simulink model "TodoModelo"  (R2020b)
settings: Solver=VariableStepAuto  StartTime=0.0  StopTime=10.0  RelTol=1e-3
values from neighbouring files (symbols this model uses):
  delay = exp(-ts*s/2)    [ControlP.m]
  Fa = tf(1,1)    [ControlP.m]
  K = mu*Kp    [ControlP.m]    (also in ControlPID_RF.m)
  P = Km/(Tm*s+1)/(Tf*s+1)    [ControlP.m]    (also in ControlPID_RF.m)
  Pd = c2d(P,ts)    [ControlP.m]    (also in ControlPID_RF.m = -P)
  ts = 0.005    [ControlP.m]    (also in ControlPID_RF.m; DatosIdentVel_rampa.mat)
  Ts = ts    (= 0.005)    [ControlP.m]
settings Model: Creator=Fran  LastModifiedBy=Fran

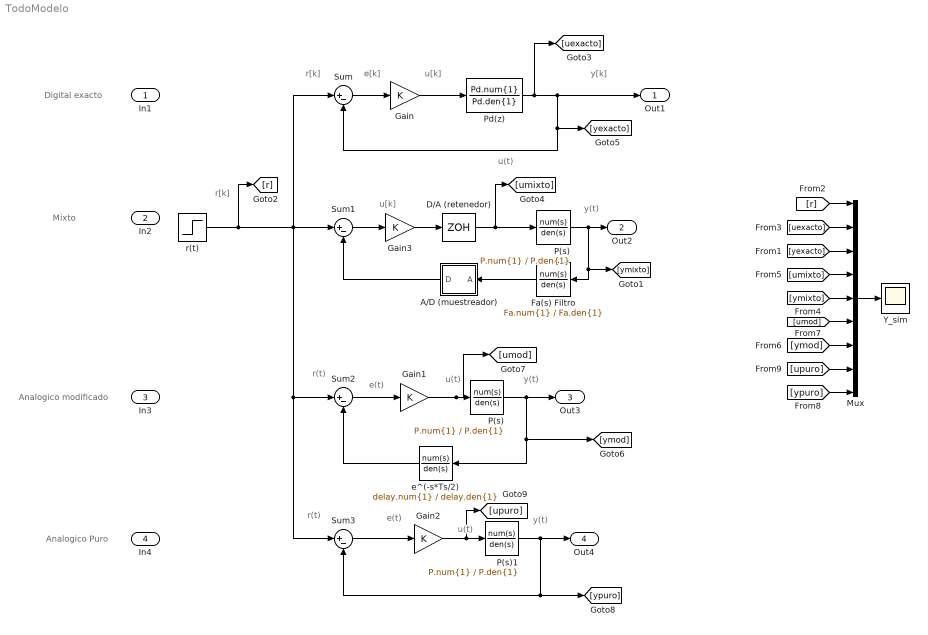
== system TodoModelo ==
  note: Analogico Puro
  note: Analogico modificado
  note: Mixto
  note: Digital exacto
  note: e[k]
  note: r[k]
  note: y[k]
  note: u[k]
  note: y(t)
  note: u[k]
  note: r[k]
  note: u(t)
  note: u(t)
  note: r(t)
  note: y(t)
  note: e(t)
  note: y(t)
  note: r(t)
  note: u(t)
  note: e(t)
  In1 : Inport
  In2 : Inport  Port=2
  In3 : Inport  Port=3
  In4 : Inport  Port=4
  A/D (muestreador) : Subsystem
  D/A (retenedor) : ZeroOrderHold  SampleTime=ts
  Fa(s) Filtro : TransferFcn  Numerator=Fa.num{1}  Denominator=Fa.den{1}
  Gain{,1..3} (4 alike) : Gain  Gain=K
  Mux : Mux  Inputs=9
  P(s) : TransferFcn  Numerator=P.num{1}  Denominator=P.den{1}
  "P(s) " : TransferFcn  Numerator=P.num{1}  Denominator=P.den{1}
  P(s)1 : TransferFcn  Numerator=P.num{1}  Denominator=P.den{1}
  Pd(z) : DiscreteTransferFcn  Numerator=Pd.num{1}  Denominator=Pd.den{1}  SampleTime=Ts
  Sum{,1..3} (4 alike) : Sum  Inputs=|+-
  Y_sim : Scope
  e^(-s*Ts/2) : TransferFcn  Numerator=delay.num{1}  Denominator=delay.den{1}
  r(t) : Step  SampleTime=ts
  Out1 : Outport
  Out2 : Outport  Port=2
  Out3 : Outport  Port=3
  Out4 : Outport  Port=4
  wires:
  Sum/1 -> Gain/1
  Gain/1 -> Pd(z)/1
  Mux/1 -> Y_sim/1
  Fa(s) Filtro/1 -> A/D (muestreador)/1(A)
  D/A (retenedor)/1 -> [umixto], "P(s) "/1
  [r] -> Mux/1
  "P(s) "/1 -> Fa(s) Filtro/1, [ymixto], Out2/1
  r(t)/1 -> Sum1/1, Sum/1, Sum3/1, Sum2/1, [r]
  [yexacto] -> Mux/3
  [uexacto] -> Mux/2
  Sum2/1 -> Gain1/1
  e^(-s*Ts/2)/1 -> Sum2/2
  P(s)/1 -> [ymod], e^(-s*Ts/2)/1, Out3/1
  Gain1/1 -> [umod], P(s)/1
  P(s)1/1 -> [ypuro], Sum3/2, Out4/1
  Gain2/1 -> [upuro], P(s)1/1
  Sum3/1 -> Gain2/1
  A/D (muestreador)/1(D) -> Sum1/2
  Sum1/1 -> Gain3/1
  Gain3/1 -> D/A (retenedor)/1
  Pd(z)/1 -> [uexacto], Sum/2, [yexacto], Out1/1
  [umixto] -> Mux/4
  [ymixto] -> Mux/5
  [umod] -> Mux/6
  [ymod] -> Mux/7
  [upuro] -> Mux/8
  [ypuro] -> Mux/9

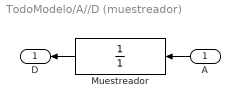
== system TodoModelo/A//D (muestreador) ==
  A : Inport
  Muestreador : DiscreteTransferFcn  Numerator=1  Denominator=1  SampleTime=ts
  D : Outport
  wires:
  A/1 -> Muestreador/1
  Muestreador/1 -> D/1
